simulink model "rocketdynamics"  (R2024b)
settings: Solver=VariableStepAuto  StartTime=0.0  StopTime=10.0  RelTol=1e-3
undefined symbols (not defined in the file or in its folder): AMB, MSL, SIM
settings Model: Creator=Leonardo Perina  LastModifiedBy=Leonardo Perina

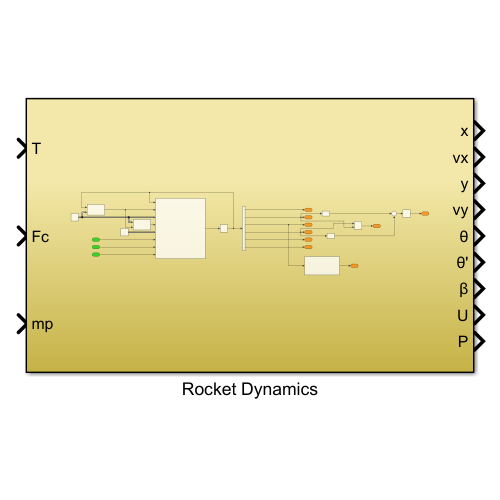
[thumbnail: Simulink's stored preview of the top-level diagram]
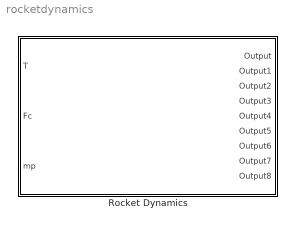
== system rocketdynamics ==
  Rocket Dynamics : Subsystem

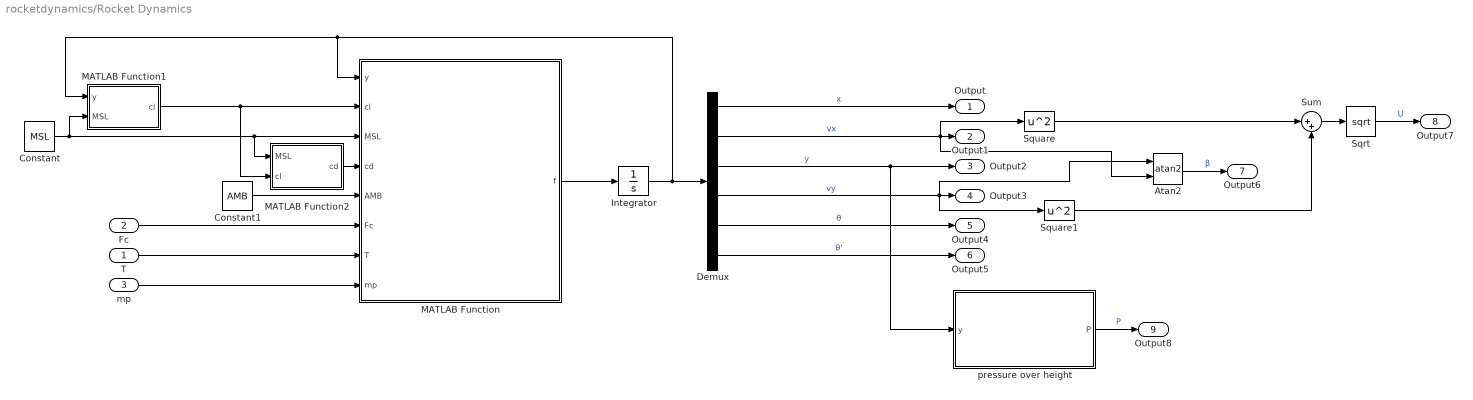
== system rocketdynamics/Rocket Dynamics ==
  T : Inport
  Fc : Inport  Port=2
  mp : Inport  Port=3
  Atan2 : Trigonometry  Operator=atan2
  Constant : Constant  Value=MSL  OutDataTypeStr=Bus: MSLbus
  Constant1 : Constant  Value=AMB  OutDataTypeStr=Bus: AMBbus
  Demux : Demux  Outputs=6
  Integrator : Integrator  InitialCondition=SIM.y0_sim
  MATLAB Function : MATLAB Function  TreatAsAtomicUnit=on
  MATLAB Function1 : MATLAB Function  TreatAsAtomicUnit=on
  MATLAB Function2 : MATLAB Function  TreatAsAtomicUnit=on
  Sqrt : Sqrt
  Square : Math  Operator=square
  Square1 : Math  Operator=square
  Sum : Sum  Inputs=|++
  pressure over height : Subsystem
  Output : Outport
  Output1 : Outport  Port=2
  Output2 : Outport  Port=3
  Output3 : Outport  Port=4
  Output4 : Outport  Port=5
  Output5 : Outport  Port=6
  Output6 : Outport  Port=7
  Output7 : Outport  Port=8
  Output8 : Outport  Port=9
  wires:
  mp/1 -> MATLAB Function/8(mp)
  T/1 -> MATLAB Function/7(T)
  Fc/1 -> MATLAB Function/6(Fc)
  Constant1/1 -> MATLAB Function/5(AMB)
  Constant/1 -> MATLAB Function2/1(MSL), MATLAB Function/3(MSL), MATLAB Function1/2(MSL)
  MATLAB Function/1(f) -> Integrator/1
  Integrator/1 -> Demux/1, MATLAB Function/1(y), MATLAB Function1/1(y)
  MATLAB Function1/1(cl) -> MATLAB Function2/2(cl), MATLAB Function/2(cl)
  MATLAB Function2/1(cd) -> MATLAB Function/4(cd)
  Demux/1 -> Output/1  "x"
  Demux/2 -> Square/1, Atan2/2, Output1/1  "vx"
  Demux/3 -> pressure over height/1(y), Output2/1  "y"
  Demux/4 -> Square1/1, Atan2/1, Output3/1  "vy"
  Demux/5 -> Output4/1  "θ"
  Demux/6 -> Output5/1  "θ'"
  Atan2/1 -> Output6/1  "β"
  Sqrt/1 -> Output7/1  "U"
  Sum/1 -> Sqrt/1
  Square/1 -> Sum/1
  Square1/1 -> Sum/2
  pressure over height/1(P) -> Output8/1  "P"

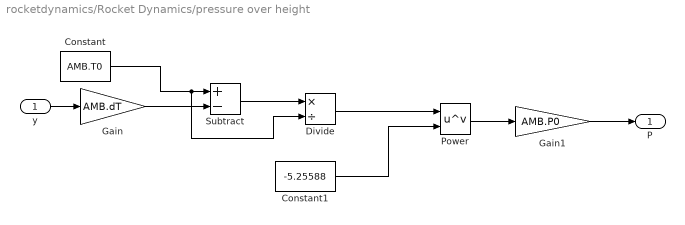
== system rocketdynamics/Rocket Dynamics/pressure over height ==
  y : Inport
  Constant : Constant  Value=AMB.T0
  Constant1 : Constant  Value=-5.25588
  Divide : Product  Inputs=*/
  Gain : Gain  Gain=AMB.dT
  Gain1 : Gain  Gain=AMB.P0
  Power : Math  Operator=pow
  Subtract : Sum  Inputs=+-
  P : Outport
  wires:
  Constant/1 -> Divide/2, Subtract/1
  y/1 -> Gain/1
  Gain/1 -> Subtract/2
  Subtract/1 -> Divide/1
  Divide/1 -> Power/1
  Constant1/1 -> Power/2
  Power/1 -> Gain1/1
  Gain1/1 -> P/1

== matlab function rocketdynamics/Rocket Dynamics/MATLAB Function1 ==
  data: y input; cl output; MSL input
function cl = fcn(y, MSL)


th = y(5);
cl = ...
    (th > MSL.thlim(2) & th <= MSL.thlim(3)) .* MSL.clt.*th + ...
    (th > MSL.thlim(3) & th <= MSL.thlim(4)) .* ...
    (MSL.clts.*(th - MSL.thlim(3)) + MSL.clt.*MSL.thlim(3)) + ...
    (th >= MSL.thlim(1) & th < MSL.thlim(2)) .* ...
    (MSL.clts.*(th - MSL.thlim(2)) + MSL.clt.*MSL.thlim(2));

== matlab function rocketdynamics/Rocket Dynamics/MATLAB Function ==
  data: f output; y input; cl input; MSL input; cd input; AMB input; Fc input; T input; mp input
function f  = validation_model_variablemassNrho(y, cl, MSL, cd, AMB, Fc, T, mp)
%VALIDATION_MODEL_VARIABLEMASSNRHO it is a translation in Simulink of the
%equivalent function


g = AMB.g0;

% xp   = y(1);
vx   = y(2);
yp   = y(3);
vy   = y(4);
th   = y(5);
thd  = y(6);
% mp   = y(7);
beta = atan2(vy,vx);
U2   = vx^2 + vy^2;
% cl   = MSLfnc.cl(th);
% cd   = MSLfnc.cd(th);

rho = 1.225*(1 + AMB.lambda*yp/AMB.T0).^(-AMB.g0/(AMB.R*AMB.lambda));

m = MSL.ms + mp;


f = zeros(6, 1);
% if mp > 0
%     f(7) = MSL.mdot;
%     T = MSL.T;
% else
%     f(7) = 0;
%     T = 0;
% end

f(1) = vx;
f(3) = vy;
f(5) = thd;

Fa   = 0.5 * rho * U2 * MSL.l * MSL.diam;

f(2) = ( -Fc*sin( beta + th ) + T*cos( beta + th ) + ...
    Fa * (-cl*sin(beta) - cd*cos(beta))) * 1/m;
f(4) = (  Fc*cos( beta + th ) + T*sin( beta + th ) + ...
    Fa * (cl*cos(beta)  - cd*sin(beta))) * 1/m - g;
f(6) = (-Fc*MSL.lc - Fa*(cl*cos(th) + cd*sin(th))*MSL.la - MSL.thc*thd) * 1/MSL.J;


end

== matlab function rocketdynamics/Rocket Dynamics/MATLAB Function2 ==
  data: MSL input; cl input; cd output
function cd = fcn(MSL, cl)

cd =  MSL.cd0 + MSL.k*cl^2;
